simulink model "EKF"  (R2021b)
settings: Solver=ode4  StartTime=0.0  StopTime=200  FixedStep=0.02  RelTol=1e-3
libraries: commchan3 x2
(part 1 of 4)
settings Model: Creator=12406  LastModifiedBy=aryal
settings SolverCC: AlgebraicLoopSolver=TrustRegion

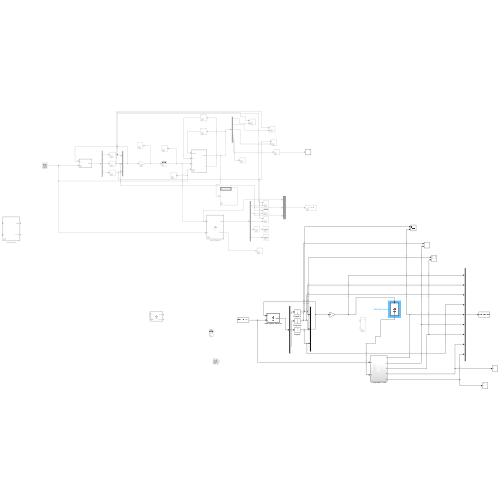
[thumbnail: Simulink's stored preview of the top-level diagram]
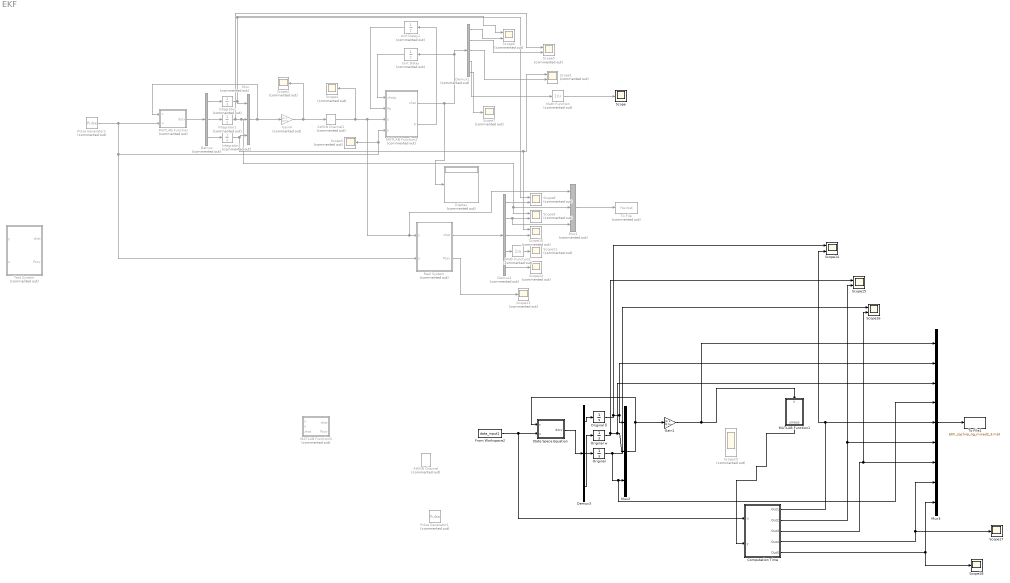
== system EKF ==
  AWGN Channel : commchan3/AWGN Channel  Commented=on  InputProcessing=Columns as channels (frame based)  seed=65  noiseMode=Variance from mask  EbNodB=10  EsNodB=10  SNRdB=10  bitsPerSym=1  Ps=1  Tsym=1  variance=1e-6
  AWGN Channel1 : commchan3/AWGN Channel  Commented=on  InputProcessing=Columns as channels (frame based)  seed=65  noiseMode=Variance from mask  EbNodB=10  EsNodB=10  SNRdB=65  bitsPerSym=1  Ps=1  Tsym=1  variance=1e-6
  Computation Time : Subsystem
  Demux : Demux  Commented=on  Outputs=3
  Demux1 : Demux  Commented=on  Outputs=5
  Demux2 : Demux  Commented=on  Outputs=5
  Demux3 : Demux  Outputs=3
  Display : Display  Commented=on
  From Workspace2 : FromWorkspace  VariableName=data_input1  SampleTime=0.02
  Gain1 : Gain  Gain=[0, 1, 0]  Multiplication=Matrix(K*u)
  Gain4 : Gain  Commented=on  Gain=[0, 1, 0]  Multiplication=Matrix(K*u)
  Integrator : Integrator  Commented=on
  Integrator1 : Integrator  Commented=on
  Integrator3 : Integrator  Commented=on
  MATLAB Function : MATLAB Function  Commented=on  TreatAsAtomicUnit=on
  MATLAB Function1 : MATLAB Function  TreatAsAtomicUnit=on
  MATLAB Function2 : MATLAB Function  Commented=on  TreatAsAtomicUnit=on  SystemSampleTime=0.02
  MATLAB Function3 : MATLAB Function  Commented=on  TreatAsAtomicUnit=on
  Math Function : Math  Commented=on  Operator=reciprocal  SaturateOnIntegerOverflow=on
  Math Function1 : Math  Commented=on  Operator=reciprocal  SaturateOnIntegerOverflow=on
  Mux : Mux  Commented=on  Inputs=3
  Mux1 : Mux  Commented=on  Inputs=3
  Mux2 : Mux  Inputs=3
  Mux3 : Mux  Inputs=9
  "Original " : Integrator
  Original w : Integrator
  "Original δ " : Integrator
  Pulse Generator1 : DiscretePulseGenerator  Commented=on  PulseType=Time based  Amplitude=0.2  PulseWidth=50
  Pulse Generator2 : DiscretePulseGenerator  Commented=on  PulseType=Time based  Amplitude=0.1  PulseWidth=50
  Real System : MATLAB Function  Commented=on  TreatAsAtomicUnit=on  SystemSampleTime=0.02
  Scope : Scope
  Scope{1,5..6,8..10,20} (7 alike) : Scope  Commented=on  NumInputPorts=2
  Scope{2..4,7,11..13} (7 alike) : Scope  Commented=on
  Scope14 : Scope  NumInputPorts=2
  Scope15 : Scope  NumInputPorts=2
  Scope16 : Scope  NumInputPorts=2
  Scope17 : Scope
  Scope18 : Scope
  State Space Equation : MATLAB Function  TreatAsAtomicUnit=on
  Test System : MATLAB Function  Commented=on  TreatAsAtomicUnit=on  SystemSampleTime=0.02
  To File : ToFile  Commented=on  Filename=fre.mat  MatrixName=f
  To File1 : ToFile  Filename=EKF_sqchirp_ng_mixed2_3.mat  MatrixName=w  SampleTime=0.02
  Unit Delay : UnitDelay  Commented=on  InitialCondition=[0.01;0.01;0.01;1/3.5;2]  SampleTime=0.02  HasFrameUpgradeWarning=on
  Unit Delay1 : UnitDelay  Commented=on  InitialCondition=ones(25,1)*1e2  SampleTime=0.02  HasFrameUpgradeWarning=on
  wires:
  Demux1/1 -> Scope6/2
  Integrator/1 -> Scope8/1, Scope6/1, Mux/1
  Demux1/5 -> Scope7/1
  Demux1/4 -> Math Function/1
  Integrator1/1 -> Mux1/2, Scope9/1, Mux/2, Scope5/1
  Unit Delay/1 -> MATLAB Function2/1(xhatp)
  Demux/3 -> Integrator3/1
  MATLAB Function/1(dotx) -> Demux/1
  Gain4/1 -> AWGN Channel1/1, Scope2/1
  Demux1/2 -> Scope5/2
  Demux/2 -> Integrator1/1
  MATLAB Function2/2(P) -> Unit Delay1/1
  Unit Delay1/1 -> MATLAB Function2/2(Pp)
  Integrator3/1 -> Scope10/1, Scope1/1, Mux/3
  Demux/1 -> Integrator/1
  Mux/1 -> Gain4/1, MATLAB Function/1(x)
  MATLAB Function2/1(xhat) -> Display/1, Demux1/1, Unit Delay/1
  Demux1/3 -> Scope1/2
  Pulse Generator2/1 -> Real System/2(u), Scope3/1, MATLAB Function2/4(u), MATLAB Function/2(u)
  Math Function/1 -> Scope/1
  Real System/1(xhat) -> Demux2/1
  Demux2/1 -> Scope8/2
  Demux2/2 -> Mux1/3, Scope9/2
  Demux2/3 -> Scope10/2
  Demux2/4 -> Math Function1/1
  Demux2/5 -> Scope12/1
  Math Function1/1 -> Scope11/1
  Real System/2(Pcov) -> Scope13/1
  Mux1/1 -> To File/1
  AWGN Channel1/1 -> Mux1/1, Real System/1(y), MATLAB Function2/3(y), Scope4/1
  "Original "/1 -> Scope16/1, Mux3/4, Mux2/3
  Demux3/2 -> Original w/1
  Original w/1 -> Scope15/1, Mux3/3, Mux2/2
  "Original δ "/1 -> Scope14/1, Mux3/2, Mux2/1
  State Space Equation/1(dotx) -> Demux3/1
  From Workspace2/1 -> Computation Time/1(u), State Space Equation/2(u)
  Demux3/1 -> "Original δ "/1
  Mux2/1 -> Gain1/1, State Space Equation/1(x)
  Demux3/3 -> "Original "/1
  Gain1/1 -> MATLAB Function1/1(y), Mux3/1
  MATLAB Function1/1(ymeas) -> Computation Time/2(y)
  Computation Time/1(Out1) -> Mux3/5, Scope14/2
  Computation Time/2(Out2) -> Scope15/2, Mux3/6
  Computation Time/3(Out3) -> Scope16/2, Mux3/7
  Computation Time/4(Out4) -> Scope17/1, Mux3/8
  Computation Time/5(Out5) -> Scope18/1, Mux3/9
  Mux3/1 -> To File1/1

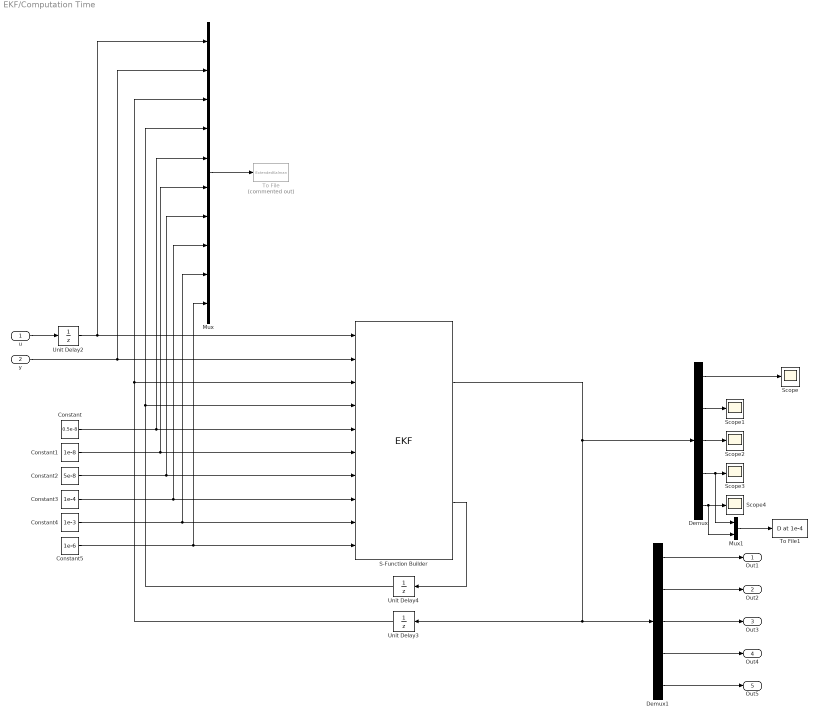
== system EKF/Computation Time ==
  u : Inport
  y : Inport  Port=2
  Constant : Constant  Value=0.5e-8
  Constant1 : Constant  Value=1e-8
  Constant2 : Constant  Value=5e-8
  Constant3 : Constant  Value=1e-4
  Constant4 : Constant  Value=1e-3
  Constant5 : Constant  Value=1e-6
  Demux : Demux  Outputs=5
  Demux1 : Demux  Outputs=5
  Mux : Mux  Inputs=10
  Mux1 : Mux  Inputs=2
  S-Function Builder : S-Function  FunctionName=EKF  SFunctionModules=EKF_wrapper EKF_Code EKF_Code_Call  SFunctionDeploymentMode=off  EnableBusSupport=off  mask(S-Function Builder){}
      mask help: Simulink:masks:SFunctionBuilder_MD
      mask init:
      | val = [[.9  0.75 0.75 1 1 .9 .9 1]',[1 1 0.75 0.75 .9 .9 1 .9]'];try , sys = get_param(gcb,'SfunBuilderFcnName');if isempty(sys), sys = get_param(gcb,'FunctionName'); end,catch, sys = get_param(gcb,'FunctionName'); end
      settings: CopyFcn=set_param(gcbh,'LinkStatus','none')  OpenFcn=sfunctionwizard(gcbh)
      mask Display: plot(val(:,1),val(:,2)),disp(sys),port_label('input',1,'u'),port_label('input',2,'y'),port_label('input',3,'xhatp'),port_label('input',4,'Pkp'),port_label('input',5,'Q11'),port_label('input',6,'Q22'),port_label('input',7,'Q33'),port_label('input',8,'Q44'),port_label('input',9,'Q55'),port_label('input',10,'R'),port_label('output',1,'xhat'),port_label('output',2,'Pk')
  Scope{,1..4} (5 alike) : Scope
  To File : ToFile  Commented=on  Filename=ExtendedKalman  SampleTime=0.02
  To File1 : ToFile  Filename=D at 1e-4  SampleTime=0.02
  Unit Delay2 : UnitDelay  SampleTime=0.02  HasFrameUpgradeWarning=on
  Unit Delay3 : UnitDelay  InitialCondition=[0;0;0;2;2]  SampleTime=0.02  HasFrameUpgradeWarning=on
  Unit Delay4 : UnitDelay  InitialCondition=reshape(diag([10, 10, 10, 10, 10]), 25, 1)  SampleTime=0.02  HasFrameUpgradeWarning=on
  Out1 : Outport
  Out2 : Outport  Port=2
  Out3 : Outport  Port=3
  Out4 : Outport  Port=4
  Out5 : Outport  Port=5
  wires:
  y/1 -> Mux/2, S-Function Builder/2
  S-Function Builder/1 -> Demux/1, Demux1/1, Unit Delay3/1
  Constant2/1 -> Mux/7, S-Function Builder/7
  u/1 -> Unit Delay2/1
  Constant4/1 -> Mux/9, S-Function Builder/9
  Unit Delay3/1 -> Mux/3, S-Function Builder/3
  Constant3/1 -> Mux/8, S-Function Builder/8
  Constant1/1 -> Mux/6, S-Function Builder/6
  Constant/1 -> Mux/5, S-Function Builder/5
  Unit Delay4/1 -> Mux/4, S-Function Builder/4
  Constant5/1 -> Mux/10, S-Function Builder/10
  Unit Delay2/1 -> Mux/1, S-Function Builder/1
  S-Function Builder/2 -> Unit Delay4/1
  Demux/1 -> Scope/1
  Demux/2 -> Scope1/1
  Demux/3 -> Scope2/1
  Demux/5 -> Mux1/2, Scope4/1
  Demux/4 -> Mux1/1, Scope3/1
  Mux/1 -> To File/1
  Demux1/2 -> Out2/1
  Demux1/1 -> Out1/1
  Demux1/3 -> Out3/1
  Demux1/4 -> Out4/1
  Demux1/5 -> Out5/1
  Mux1/1 -> To File1/1

== matlab function EKF/Test System ==
  data: y input; xhat output; u input; Pcov output
function [xhat, Pcov]= fcn(y, u)
    Ts = 0.02;
    Qk = eye(5);
    Qk(1,1) = 1e-7;
    Qk(2,2) = 1e-7;
    Qk(3,3) = 1e-7;
    Qk(4,4) = 1e-5;
    Qk(5,5) = 1e-2;
    Rk = 1e-6;
    C = [0, 1, 0, 0, 0];
    
    persistent xhat_p Pcov_p;
    
    if isempty(xhat_p)
        xhat_p = [0;0;0;1/2;4];
        Pcov_p = 1000*ones(5, 5);
    end
    
    xkm = Fd(xhat_p, u, Ts);
    Fk = J_wrtX(xhat_p, u, Ts);
    Pkm = Fk*Pcov_p*Fk' + Qk;
    
    y_err = y - C*xkm;
    Sk = C*Pkm*C' + Rk;
    Kk = Pkm * C'*inv(Sk);
    xhat = xkm + Kk*y_err;
    Pcov_final = (eye(5) - Kk*C)*Pkm;
    
    Pcov = reshape(Pcov_final, [25, 1]);
    
    xhat_p = xhat;
    Pcov_p = Pcov_final;

    function X1 = Fd(x, u, Ts)
        x1 = x(1);
        x2 = x(2);
        x3 = x(3);
        M = x(4);
        D = x(5);
        X1 = [x1 + (Ts*(6*x2 + Ts*x3 + Ts*(x3 - (Ts*(5*M*u + (x2 + (Ts*x3)/2)*(100*M + 5*D*M) + 100*M*(x1 + (Ts*x2)/2) + (x3 - (Ts*(5*M*u + 100*M*x1 + x3*(D*M + 5) + x2*(100*M + 5*D*M)))/2)*(D*M + 5)))/2) + Ts*(x3 - (Ts*(5*M*u + 100*M*x1 + x3*(D*M + 5) + x2*(100*M + 5*D*M)))/2)))/6;                                                                                                                                          
            x2 - (Ts*(Ts*(5*M*u + (x2 + (Ts*x3)/2)*(100*M + 5*D*M) + 100*M*(x1 + (Ts*x2)/2) + (x3 - (Ts*(5*M*u + 100*M*x1 + x3*(D*M + 5) + x2*(100*M + 5*D*M)))/2)*(D*M + 5)) - 6*x3 + Ts*((x2 + (Ts*(x3 - (Ts*(5*M*u + 100*M*x1 + x3*(D*M + 5) + x2*(100*M + 5*D*M)))/2))/2)*(100*M + 5*D*M) + 5*M*u + 100*M*(x1 + (Ts*(x2 + (Ts*x3)/2))/2) + (D*M + 5)*(x3 - (Ts*(5*M*u + (x2 + (Ts*x3)/2)*(100*M + 5*D*M) + 100*M*(x1 + (Ts*x2)/2) + (x3 - (Ts*(5*M*u + 100*M*x1 + x3*(D*M + 5) + x2*(100*M + 5*D*M)))/2)*(D*M + 5)))/2)) + Ts*(5*M*u + 100*M*x1 + x3*(D*M + 5) + x2*(100*M + 5*D*M))))/6;
            x3 - (Ts*(2*(x2 + (Ts*(x3 - (Ts*(5*M*u + 100*M*x1 + x3*(D*M + 5) + x2*(100*M + 5*D*M)))/2))/2)*(100*M + 5*D*M) + 30*M*u + 100*M*x1 + x3*(D*M + 5) + 200*M*(x1 + (Ts*(x2 + (Ts*x3)/2))/2) + 2*(x2 + (Ts*x3)/2)*(100*M + 5*D*M) + 2*(D*M + 5)*(x3 - (Ts*(5*M*u + (x2 + (Ts*x3)/2)*(100*M + 5*D*M) + 100*M*(x1 + (Ts*x2)/2) + (x3 - (Ts*(5*M*u + 100*M*x1 + x3*(D*M + 5) + x2*(100*M + 5*D*M)))/2)*(D*M + 5)))/2) + 200*M*(x1 + (Ts*x2)/2) + (x3 - Ts*((x2 + (Ts*(x3 - (Ts*(5*M*u + 100*M*x1 + x3*(D*M + 5) + x2*(100*M + 5*D*M)))/2))/2)*(100*M + 5*D*M) + 5*M*u + 100*M*(x1 + (Ts*(x2 + (Ts*x3)/2))/2) + (D*M + 5)*(x3 - (Ts*(5*M*u + (x2 + (Ts*x3)/2)*(100*M + 5*D*M) + 100*M*(x1 + (Ts*x2)/2) + (x3 - (Ts*(5*M*u + 100*M*x1 + x3*(D*M + 5) + x2*(100*M + 5*D*M)))/2)*(D*M + 5)))/2)))*(D*M + 5) + x2*(100*M + 5*D*M) + 2*(x3 - (Ts*(5*M*u + 100*M*x1 + x3*(D*M + 5) + x2*(100*M + 5*D*M)))/2)*(D*M + 5) + (x2 + Ts*(x3 - (Ts*(5*M*u + (x2 + (Ts*x3)/2)*(100*M + 5*D*M) + 100*M*(x1 + (Ts*x2)/2) + (x3 - (Ts*(5*M*u + 100*M*x1 + x3*(D*M + 5) + x2*(100*M + 5*D*M)))/2)*(D*M + 5)))/2))*(100*M + 5*D*M) + 100*M*(x1 + Ts*(x2 + (Ts*(x3 - (Ts*(5*M*u + 100*M*x1 + x3*(D*M + 5) + x2*(100*M + 5*D*M)))/2))/2))))/6;
              M;
              D];
    end

    function Ad = J_wrtX(x, u, Ts)
        x1 = x(1);
        x2 = x(2);
        x3 = x(3);
        M = x(4);
        D = x(5);
        Ad = [ 1 - (Ts*(50*M*Ts^2 + (Ts^2*(100*M - 50*M*Ts*(D*M + 5)))/2))/6,                                                                                                                                                                                                                                                                                                                                                                                     -(Ts*((Ts^2*(100*M + 5*D*M))/2 + (Ts^2*(100*M + 50*M*Ts + 5*D*M - (Ts*(D*M + 5)*(100*M + 5*D*M))/2))/2 - 6))/6,                                                                                                                                                                                                                                                                                                                                                                                                                (Ts*(Ts - Ts*((Ts*(D*M + 5))/2 - 1) + Ts*((Ts*((D*M + 5)*((Ts*(D*M + 5))/2 - 1) - (Ts*(100*M + 5*D*M))/2))/2 + 1)))/6,                                                                                                                                                                                                                                                                                                                                                                                                                                                                                                                                                                                                                                                                                                                                                                                                                                                                                                                                                                                                                                                                                                                                                                                                                                                                                                                                                                                                                                                                                                                                                                                                                                                                                                                                                                                                                                                                                                                                                                                                                                                                                   -(Ts*((Ts^2*(5*u + 100*x1 + D*x3 + x2*(5*D + 100)))/2 + (Ts^2*(5*u + 100*x1 + 50*Ts*x2 + (5*D + 100)*(x2 + (Ts*x3)/2) + D*(x3 - (Ts*(5*M*u + 100*M*x1 + x3*(D*M + 5) + x2*(100*M + 5*D*M)))/2) - (Ts*(D*M + 5)*(5*u + 100*x1 + D*x3 + x2*(5*D + 100)))/2))/2))/6,                                                                                                                                                                                                                                                                                                                                                                                                                                                                                                                                                                                                                                                                                                                                                                                                                                                                                                                                                                                                                                                                                                                                                                                                                                                                                                                                                                                                                                                                                                                                                                                                                                                        -(Ts*((Ts^2*(5*M*(x2 + (Ts*x3)/2) + M*(x3 - (Ts*(5*M*u + 100*M*x1 + x3*(D*M + 5) + x2*(100*M + 5*D*M)))/2) - (Ts*(D*M + 5)*(5*M*x2 + M*x3))/2))/2 + (Ts^2*(5*M*x2 + M*x3))/2))/6;
                                                                                                                                               -(Ts*(100*M*Ts + Ts*(100*M - 50*M*Ts*(D*M + 5)) - Ts*(25*M*Ts^2*(100*M + 5*D*M) - 100*M + (Ts*(D*M + 5)*(100*M - 50*M*Ts*(D*M + 5)))/2)))/6,                                                                                                                                                                                                                                                  1 - (Ts*(Ts*(100*M + 5*D*M) + Ts*(100*M + 50*M*Ts + 5*D*M - (Ts*(D*M + 5)*(100*M + 5*D*M))/2) - Ts*(((Ts^2*(100*M + 5*D*M))/4 - 1)*(100*M + 5*D*M) - 50*M*Ts + (Ts*(D*M + 5)*(100*M + 50*M*Ts + 5*D*M - (Ts*(D*M + 5)*(100*M + 5*D*M))/2))/2)))/6,                                                                                                                                                                                                                                                                                    -(Ts*(Ts*(D*M + 5) + Ts*(25*M*Ts^2 + ((Ts*((D*M + 5)*((Ts*(D*M + 5))/2 - 1) - (Ts*(100*M + 5*D*M))/2))/2 + 1)*(D*M + 5) - (Ts*((Ts*(D*M + 5))/2 - 1)*(100*M + 5*D*M))/2) - Ts*((D*M + 5)*((Ts*(D*M + 5))/2 - 1) - (Ts*(100*M + 5*D*M))/2) - 6))/6,                                                                                                                                                                                                                                                                                                                                                                                                                                                                                                                                                                                                                                                                                                                                                                                                                                                                                                                                                                                                                                                                                                                                                                                                                                                                                                                                                                                                                                                                                         -(Ts*(Ts*(5*u + 100*x1 + 50*Ts*x2 + (5*D + 100)*(x2 + (Ts*x3)/2) + D*(x3 - (Ts*(5*M*u + 100*M*x1 + x3*(D*M + 5) + x2*(100*M + 5*D*M)))/2) - (Ts*(D*M + 5)*(5*u + 100*x1 + D*x3 + x2*(5*D + 100)))/2) + Ts*(5*u + 100*x1 + (5*D + 100)*(x2 + (Ts*(x3 - (Ts*(5*M*u + 100*M*x1 + x3*(D*M + 5) + x2*(100*M + 5*D*M)))/2))/2) + D*(x3 - (Ts*(5*M*u + (x2 + (Ts*x3)/2)*(100*M + 5*D*M) + 100*M*(x1 + (Ts*x2)/2) + (x3 - (Ts*(5*M*u + 100*M*x1 + x3*(D*M + 5) + x2*(100*M + 5*D*M)))/2)*(D*M + 5)))/2) + 50*Ts*(x2 + (Ts*x3)/2) - (Ts^2*(100*M + 5*D*M)*(5*u + 100*x1 + D*x3 + x2*(5*D + 100)))/4 - (Ts*(D*M + 5)*(5*u + 100*x1 + 50*Ts*x2 + (5*D + 100)*(x2 + (Ts*x3)/2) + D*(x3 - (Ts*(5*M*u + 100*M*x1 + x3*(D*M + 5) + x2*(100*M + 5*D*M)))/2) - (Ts*(D*M + 5)*(5*u + 100*x1 + D*x3 + x2*(5*D + 100)))/2))/2) + Ts*(5*u + 100*x1 + D*x3 + x2*(5*D + 100))))/6,                                                                                                                                                                                                                                                                                                                                                                                                                                                                                                                                                                                                                                                                                                                                                                                                                                                                                                                                                                                                                                                                                                                                                                                              -(Ts*(Ts*(5*M*(x2 + (Ts*x3)/2) + M*(x3 - (Ts*(5*M*u + 100*M*x1 + x3*(D*M + 5) + x2*(100*M + 5*D*M)))/2) - (Ts*(D*M + 5)*(5*M*x2 + M*x3))/2) + Ts*(5*M*x2 + M*x3) + Ts*(5*M*(x2 + (Ts*(x3 - (Ts*(5*M*u + 100*M*x1 + x3*(D*M + 5) + x2*(100*M + 5*D*M)))/2))/2) + M*(x3 - (Ts*(5*M*u + (x2 + (Ts*x3)/2)*(100*M + 5*D*M) + 100*M*(x1 + (Ts*x2)/2) + (x3 - (Ts*(5*M*u + 100*M*x1 + x3*(D*M + 5) + x2*(100*M + 5*D*M)))/2)*(D*M + 5)))/2) - (Ts*(D*M + 5)*(5*M*(x2 + (Ts*x3)/2) + M*(x3 - (Ts*(5*M*u + 100*M*x1 + x3*(D*M + 5) + x2*(100*M + 5*D*M)))/2) - (Ts*(D*M + 5)*(5*M*x2 + M*x3))/2))/2 - (Ts^2*(5*M*x2 + M*x3)*(100*M + 5*D*M))/4)))/6;
(Ts*(100*M*(25*M*Ts^3 - 1) - 500*M + 100*M*Ts*(D*M + 5) + 50*M*Ts^2*(100*M + 5*D*M) + Ts*(D*M + 5)*(100*M - 50*M*Ts*(D*M + 5)) + (Ts^2*(100*M - 50*M*Ts*(D*M + 5))*(100*M + 5*D*M))/2 - Ts*(D*M + 5)*(25*M*Ts^2*(100*M + 5*D*M) - 100*M + (Ts*(D*M + 5)*(100*M - 50*M*Ts*(D*M + 5)))/2)))/6, (Ts*(2*((Ts^2*(100*M + 5*D*M))/4 - 1)*(100*M + 5*D*M) - 200*M*Ts - 300*M + ((Ts^2*(100*M + 50*M*Ts + 5*D*M - (Ts*(D*M + 5)*(100*M + 5*D*M))/2))/2 - 1)*(100*M + 5*D*M) - 15*D*M + Ts*(D*M + 5)*(100*M + 5*D*M) + Ts*(D*M + 5)*(100*M + 50*M*Ts + 5*D*M - (Ts*(D*M + 5)*(100*M + 5*D*M))/2) - Ts*(D*M + 5)*(((Ts^2*(100*M + 5*D*M))/4 - 1)*(100*M + 5*D*M) - 50*M*Ts + (Ts*(D*M + 5)*(100*M + 50*M*Ts + 5*D*M - (Ts*(D*M + 5)*(100*M + 5*D*M))/2))/2) + 100*M*Ts*((Ts^2*(100*M + 5*D*M))/4 - 1)))/6, 1 - (Ts*(50*M*Ts^2 - 2*(D*M + 5)*((Ts*(D*M + 5))/2 - 1) - (D*M + 5)*(Ts*(25*M*Ts^2 + ((Ts*((D*M + 5)*((Ts*(D*M + 5))/2 - 1) - (Ts*(100*M + 5*D*M))/2))/2 + 1)*(D*M + 5) - (Ts*((Ts*(D*M + 5))/2 - 1)*(100*M + 5*D*M))/2) - 1) + Ts*(100*M + 5*D*M) + 2*((Ts*((D*M + 5)*((Ts*(D*M + 5))/2 - 1) - (Ts*(100*M + 5*D*M))/2))/2 + 1)*(D*M + 5) + D*M - Ts*((Ts*(D*M + 5))/2 - 1)*(100*M + 5*D*M) - 50*M*Ts^2*((Ts*(D*M + 5))/2 - 1) + Ts*((Ts*((D*M + 5)*((Ts*(D*M + 5))/2 - 1) - (Ts*(100*M + 5*D*M))/2))/2 + 1)*(100*M + 5*D*M) + 5))/6, -(Ts*(30*u + 600*x1 + 2*(5*D + 100)*(x2 + (Ts*(x3 - (Ts*(5*M*u + 100*M*x1 + x3*(D*M + 5) + x2*(100*M + 5*D*M)))/2))/2) + D*x3 + 100*Ts*x2 + 2*(5*D + 100)*(x2 + (Ts*x3)/2) + 100*Ts*(x2 + (Ts*(x3 - (Ts*(5*M*u + 100*M*x1 + x3*(D*M + 5) + x2*(100*M + 5*D*M)))/2))/2) + 2*D*(x3 - (Ts*(5*M*u + (x2 + (Ts*x3)/2)*(100*M + 5*D*M) + 100*M*(x1 + (Ts*x2)/2) + (x3 - (Ts*(5*M*u + 100*M*x1 + x3*(D*M + 5) + x2*(100*M + 5*D*M)))/2)*(D*M + 5)))/2) + D*(x3 - Ts*((x2 + (Ts*(x3 - (Ts*(5*M*u + 100*M*x1 + x3*(D*M + 5) + x2*(100*M + 5*D*M)))/2))/2)*(100*M + 5*D*M) + 5*M*u + 100*M*(x1 + (Ts*(x2 + (Ts*x3)/2))/2) + (D*M + 5)*(x3 - (Ts*(5*M*u + (x2 + (Ts*x3)/2)*(100*M + 5*D*M) + 100*M*(x1 + (Ts*x2)/2) + (x3 - (Ts*(5*M*u + 100*M*x1 + x3*(D*M + 5) + x2*(100*M + 5*D*M)))/2)*(D*M + 5)))/2))) + 100*Ts*(x2 + (Ts*x3)/2) + 2*D*(x3 - (Ts*(5*M*u + 100*M*x1 + x3*(D*M + 5) + x2*(100*M + 5*D*M)))/2) + x2*(5*D + 100) + (5*D + 100)*(x2 + Ts*(x3 - (Ts*(5*M*u + (x2 + (Ts*x3)/2)*(100*M + 5*D*M) + 100*M*(x1 + (Ts*x2)/2) + (x3 - (Ts*(5*M*u + 100*M*x1 + x3*(D*M + 5) + x2*(100*M + 5*D*M)))/2)*(D*M + 5)))/2)) - Ts*(D*M + 5)*(5*u + 100*x1 + (5*D + 100)*(x2 + (Ts*(x3 - (Ts*(5*M*u + 100*M*x1 + x3*(D*M + 5) + x2*(100*M + 5*D*M)))/2))/2) + D*(x3 - (Ts*(5*M*u + (x2 + (Ts*x3)/2)*(100*M + 5*D*M) + 100*M*(x1 + (Ts*x2)/2) + (x3 - (Ts*(5*M*u + 100*M*x1 + x3*(D*M + 5) + x2*(100*M + 5*D*M)))/2)*(D*M + 5)))/2) + 50*Ts*(x2 + (Ts*x3)/2) - (Ts^2*(100*M + 5*D*M)*(5*u + 100*x1 + D*x3 + x2*(5*D + 100)))/4 - (Ts*(D*M + 5)*(5*u + 100*x1 + 50*Ts*x2 + (5*D + 100)*(x2 + (Ts*x3)/2) + D*(x3 - (Ts*(5*M*u + 100*M*x1 + x3*(D*M + 5) + x2*(100*M + 5*D*M)))/2) - (Ts*(D*M + 5)*(5*u + 100*x1 + D*x3 + x2*(5*D + 100)))/2))/2) - Ts*(D*M + 5)*(5*u + 100*x1 + D*x3 + x2*(5*D + 100)) - (Ts^2*(100*M + 5*D*M)*(5*u + 100*x1 + D*x3 + x2*(5*D + 100)))/2 - 25*M*Ts^3*(5*u + 100*x1 + D*x3 + x2*(5*D + 100)) - Ts*(D*M + 5)*(5*u + 100*x1 + 50*Ts*x2 + (5*D + 100)*(x2 + (Ts*x3)/2) + D*(x3 - (Ts*(5*M*u + 100*M*x1 + x3*(D*M + 5) + x2*(100*M + 5*D*M)))/2) - (Ts*(D*M + 5)*(5*u + 100*x1 + D*x3 + x2*(5*D + 100)))/2) - (Ts^2*(100*M + 5*D*M)*(5*u + 100*x1 + 50*Ts*x2 + (5*D + 100)*(x2 + (Ts*x3)/2) + D*(x3 - (Ts*(5*M*u + 100*M*x1 + x3*(D*M + 5) + x2*(100*M + 5*D*M)))/2) - (Ts*(D*M + 5)*(5*u + 100*x1 + D*x3 + x2*(5*D + 100)))/2))/2))/6, -(Ts*(5*M*x2 + M*x3 + 5*M*(x2 + Ts*(x3 - (Ts*(5*M*u + (x2 + (Ts*x3)/2)*(100*M + 5*D*M) + 100*M*(x1 + (Ts*x2)/2) + (x3 - (Ts*(5*M*u + 100*M*x1 + x3*(D*M + 5) + x2*(100*M + 5*D*M)))/2)*(D*M + 5)))/2)) + 10*M*(x2 + (Ts*(x3 - (Ts*(5*M*u + 100*M*x1 + x3*(D*M + 5) + x2*(100*M + 5*D*M)))/2))/2) + 2*M*(x3 - (Ts*(5*M*u + (x2 + (Ts*x3)/2)*(100*M + 5*D*M) + 100*M*(x1 + (Ts*x2)/2) + (x3 - (Ts*(5*M*u + 100*M*x1 + x3*(D*M + 5) + x2*(100*M + 5*D*M)))/2)*(D*M + 5)))/2) + M*(x3 - Ts*((x2 + (Ts*(x3 - (Ts*(5*M*u + 100*M*x1 + x3*(D*M + 5) + x2*(100*M + 5*D*M)))/2))/2)*(100*M + 5*D*M) + 5*M*u + 100*M*(x1 + (Ts*(x2 + (Ts*x3)/2))/2) + (D*M + 5)*(x3 - (Ts*(5*M*u + (x2 + (Ts*x3)/2)*(100*M + 5*D*M) + 100*M*(x1 + (Ts*x2)/2) + (x3 - (Ts*(5*M*u + 100*M*x1 + x3*(D*M + 5) + x2*(100*M + 5*D*M)))/2)*(D*M + 5)))/2))) + 10*M*(x2 + (Ts*x3)/2) + 2*M*(x3 - (Ts*(5*M*u + 100*M*x1 + x3*(D*M + 5) + x2*(100*M + 5*D*M)))/2) - 25*M*Ts^3*(5*M*x2 + M*x3) - Ts*(D*M + 5)*(5*M*(x2 + (Ts*x3)/2) + M*(x3 - (Ts*(5*M*u + 100*M*x1 + x3*(D*M + 5) + x2*(100*M + 5*D*M)))/2) - (Ts*(D*M + 5)*(5*M*x2 + M*x3))/2) - (Ts^2*(100*M + 5*D*M)*(5*M*(x2 + (Ts*x3)/2) + M*(x3 - (Ts*(5*M*u + 100*M*x1 + x3*(D*M + 5) + x2*(100*M + 5*D*M)))/2) - (Ts*(D*M + 5)*(5*M*x2 + M*x3))/2))/2 - Ts*(D*M + 5)*(5*M*x2 + M*x3) - (Ts^2*(5*M*x2 + M*x3)*(100*M + 5*D*M))/2 - Ts*(D*M + 5)*(5*M*(x2 + (Ts*(x3 - (Ts*(5*M*u + 100*M*x1 + x3*(D*M + 5) + x2*(100*M + 5*D*M)))/2))/2) + M*(x3 - (Ts*(5*M*u + (x2 + (Ts*x3)/2)*(100*M + 5*D*M) + 100*M*(x1 + (Ts*x2)/2) + (x3 - (Ts*(5*M*u + 100*M*x1 + x3*(D*M + 5) + x2*(100*M + 5*D*M)))/2)*(D*M + 5)))/2) - (Ts*(D*M + 5)*(5*M*(x2 + (Ts*x3)/2) + M*(x3 - (Ts*(5*M*u + 100*M*x1 + x3*(D*M + 5) + x2*(100*M + 5*D*M)))/2) - (Ts*(D*M + 5)*(5*M*x2 + M*x3))/2))/2 - (Ts^2*(5*M*x2 + M*x3)*(100*M + 5*D*M))/4)))/6;
                                                                                                                                                                                                                                                                                          0,                                                                                                                                                                                                                                                                                                                                                                                                                                                                                                  0,                                                                                                                                                                                                                                                                                                                                                                                                                                                                                                                                    0,                                                                                                                                                                                                                                                                                                                                                                                                                                                                                                                                                                                                                                                                                                                                                                                                                                                                                                                                                                                                                                                                                                                                                                                                                                                                                                                                                                                                                                                                                                                                                                                                                                                                                                                                                                                                                                                                                                                                                                                                                                                                                                                                                                                                                                                                                                                                                  1,                                                                                                                                                                                                                                                                                                                                                                                                                                                                                                                                                                                                                                                                                                                                                                                                                                                                                                                                                                                                                                                                                                                                                                                                                                                                                                                                                                                                                                                                                                                                                                                                                                                  0;
                                                                                                                                                                                                                                                                                          0,                                                                                                                                                                                                                                                                                                                                                                                                                                                                                                  0,                                                                                                                                                                                                                                                                                                                                                                                                                                                                                                                                    0,                                                                                                                                                                                                                                                                                                                                                                                                                                                                                                                                                                                                                                                                                                                                                                                                                                                                                                                                                                                                                                                                                                                                                                                                                                                                                                                                                                                                                                                                                                                                                                                                                                                                                                                                                                                                                                                                                                                                                                                                                                                                                                                                                                                                                                                                                                                                                  0,                                                                                                                                                                                                                                                                                                                                                                                                                                                                                                                                                                                                                                                                                                                                                                                                                                                                                                                                                                                                                                                                                                                                                                                                                                                                                                                                                                                                                                                                                                                                                                                                                                                   1];
 
    end
end

== matlab function EKF/MATLAB Function ==
  data: x input; u input; dotx output
function dotx  = fcn(x, u)
    D = 1.5;
    M = 4.0;
    Tg = 0.2;
    Rp = 0.05;
    Ki=2;
   dotx=zeros(3,1);
    x1 = x(1);
    x2 = x(2);
    x3 = x(3);
    dotx = [x2;x3;-Ki/(M*Tg)*x1-(D/(M*Tg)+1/(Rp*M*Tg))*x2-(D/M+1/Tg)*x3-1/(M*Tg)*u];
